simulink model "data_collection_arm_integral"  (R2023b)
settings: Solver=VariableStepAuto  StartTime=0.0  StopTime=Tsim  RelTol=1e-3
values from neighbouring files (symbols this model uses):
  mag = 0.1    [one_link_robot_arm_integral.m]
  Ts = 0.1    [one_link_robot_arm_integral.m]
  x0 = (2*mx0).*rand(5,1)-mx0    [one_link_robot_arm_integral.m]
settings Model: Creator=pietrotesi  LastModifiedBy=zjhu_
settings SolverCC: AlgebraicLoopSolver=TrustRegion
settings DataIOCC: ReturnWorkspaceOutputs=off
settings DebuggingCC: UnconnectedInputMsg=warning  UnconnectedOutputMsg=warning  UnconnectedLineMsg=warning
settings ModelReferenceCC: EnableRefExpFcnMdlSchedulingChecks=on
settings RTWCC: DLArmComputeVersion=19.05

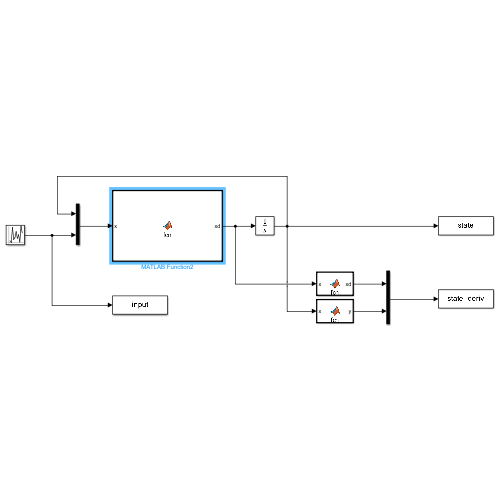
[thumbnail: Simulink's stored preview of the top-level diagram]
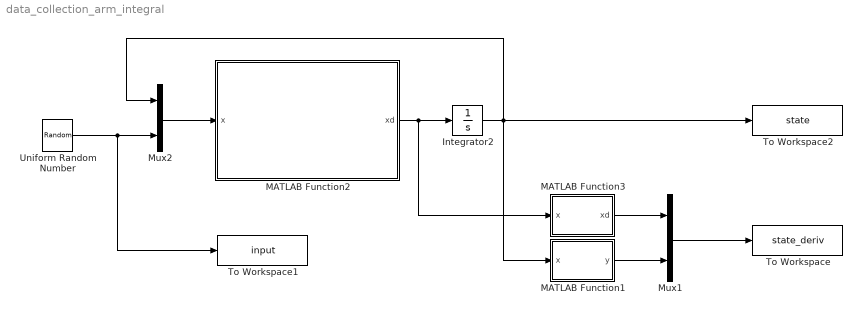
== system data_collection_arm_integral ==
  Integrator2 : Integrator  InitialCondition=x0
  MATLAB Function1 : MATLAB Function  TreatAsAtomicUnit=on
  MATLAB Function2 : MATLAB Function  TreatAsAtomicUnit=on
  MATLAB Function3 : MATLAB Function  TreatAsAtomicUnit=on
  Mux1 : Mux  Inputs=2
  Mux2 : Mux  Inputs=2
  To Workspace : ToWorkspace  VariableName=state_deriv  SaveFormat=Structure With Time  SampleTime=Ts
  To Workspace1 : ToWorkspace  VariableName=input  SaveFormat=Structure With Time  SampleTime=Ts
  To Workspace2 : ToWorkspace  VariableName=state  SaveFormat=Structure With Time  SampleTime=Ts
  Uniform Random Number : UniformRandomNumber  Minimum=-mag  Maximum=mag  SampleTime=Ts
  wires:
  Mux2/1 -> MATLAB Function2/1(x)
  MATLAB Function2/1(xd) -> MATLAB Function3/1(x), Integrator2/1
  Uniform Random Number/1 -> To Workspace1/1, Mux2/2
  Integrator2/1 -> To Workspace2/1, MATLAB Function1/1(x), Mux2/1
  Mux1/1 -> To Workspace/1
  MATLAB Function1/1(y) -> Mux1/2
  MATLAB Function3/1(xd) -> Mux1/1

== matlab function data_collection_arm_integral/MATLAB Function2 ==
  data: x input; xd output
function xd = fcn(x)
track_r = pi/3; % Track reference
noise = [0.1 0.2 0.3 0.4];
x1 = x(1);
x2 = x(2);
x3 = x(3);
x4 = x(4);
u  = x(6);

J1=0.15; J2=0.2;
F1=0.1; F2=0.15;
mas=0.4; g=9.8; d=0.1; Kc=0.4; Nc=2;

xd = [x2 + noise(1); -Kc/J2*x1 - F2/J2*x2 + Kc/J2/Nc*x3 - mas*g*d/J2*cos(x1) + noise(2);...
    x4 + noise(3); -Kc/J1/Nc*x1 + Kc/J1/Nc/Nc*x3 - F1/J1*x4 + 1/J1*u + noise(4); x1 - track_r];

== matlab function data_collection_arm_integral/MATLAB Function3 ==
  data: x input; xd output
function xd = fcn(x)

xd = x(1:4,1);

== matlab function data_collection_arm_integral/MATLAB Function1 ==
  data: x input; y output
function y = fcn(x)

y = x(1);
